simulink model "ENV_hardcoded"  (R2024b)
settings: Solver=FixedStepDiscrete  StartTime=0.0  StopTime=10.0  FixedStep=0.001  RelTol=1e-3
libraries: stm32blockslib x54, canmsglib x29, simulink x7, stm32f4xxblockslib x1
(part 2 of 5)

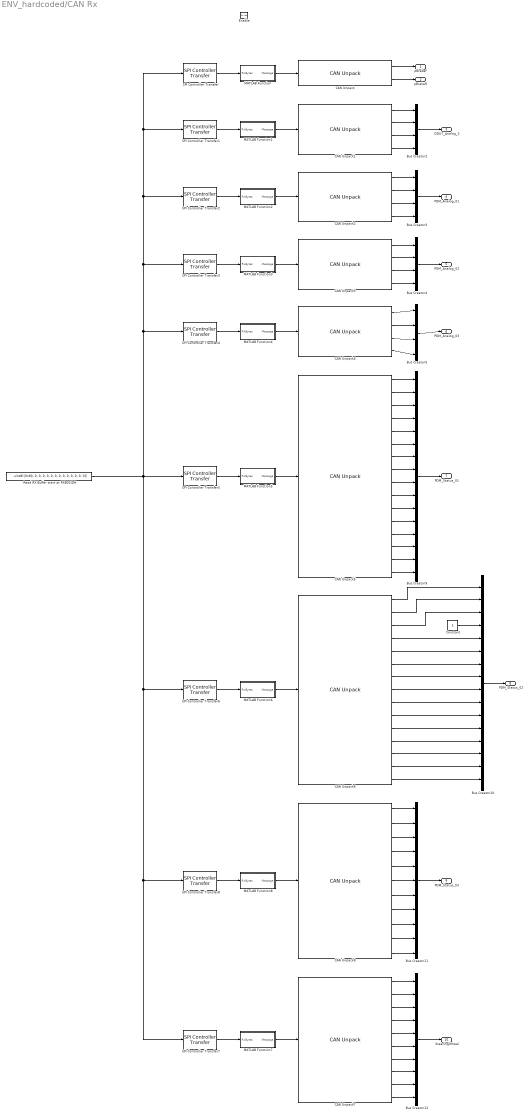
== system ENV_hardcoded/CAN Rx ==
  Enable : EnablePort
  Bus Creator10 : BusCreator  Inputs=16  OutDataTypeStr=Bus: PDM_Status_2
  Bus Creator11 : BusCreator  Inputs=11  OutDataTypeStr=Bus: PDM_Status_3
  Bus Creator12 : BusCreator  Inputs=10  OutDataTypeStr=Bus: SteeringWheelBus
  Bus Creator2 : BusCreator  Inputs=4  OutDataTypeStr=Bus: DDU7_Analoge_2
  Bus Creator3 : BusCreator  Inputs=4  OutDataTypeStr=Bus: PDM_Analoge_1
  Bus Creator4 : BusCreator  Inputs=4  OutDataTypeStr=Bus: PDM_Analoge_2
  Bus Creator5 : BusCreator  Inputs=4  OutDataTypeStr=Bus: PDM_Analoge_3
  Bus Creator9 : BusCreator  Inputs=16  OutDataTypeStr=Bus: PDM_Status_1
  CAN Unpack : canmsglib/CAN Unpack  CANdbFile=C:\Users\William\Downloads\VCUSTM32\BaselineControls\CAN\CAN3_baseline.dbc  MsgList=DDU7_Analoge_1  MsgName=DDU7_Analoge_1  MsgIDType=Standard (11-bit identifier)  MsgIdentifier=2000  MsgLength=8  SignalInfo={'pBrakeF','0','16','LE','signed','Standard','0','0.005','0','-163.84','163.835';'pBrakeR','16','16','LE','signed','Standard','0','0.005','0','-163.84','163.835'}  IDPort=off  TimestampPort=off  ErrorPort=off  RemotePort=off  LengthPort=off  StatusPort=off  ApplyMinMax=off
      settings: LibrarySourceBlock=stmutilitieslib/CAN Unpack  DataFormat=CANdb specified signals
  CAN Unpack1 : canmsglib/CAN Unpack  CANdbFile=C:\Users\William\Downloads\VCUSTM32\BaselineControls\CAN\CAN3_baseline.dbc  MsgList=DDU7_Analoge_2  MsgName=DDU7_Analoge_2  MsgIDType=Standard (11-bit identifier)  MsgIdentifier=2001  MsgLength=8  SignalInfo={'NDisplayNumberDDU7','48','8','LE','unsigned','Standard','0','1','0','0','255';'VSteeringAngle','32','16','LE','unsigned','Standard','0','0.1','0','0','6553.5';'VThrottlePedal1','0','16','LE','unsigned','Standard','0','0.1','0','0','6553.5';'VThrottlePedal2','16','16','LE','unsigned','Standard','0','0.1','0','0','6553.5'}  IDPort=off  TimestampPort=off  ErrorPort=off  RemotePort=off  LengthPort=off  StatusPort=off  ApplyMinMax=off
      settings: LibrarySourceBlock=stmutilitieslib/CAN Unpack  DataFormat=CANdb specified signals
  CAN Unpack2 : canmsglib/CAN Unpack  CANdbFile=C:\Users\William\Downloads\VCUSTM32\BaselineControls\CAN\CAN3_baseline.dbc  MsgList=PDM_Analog_01  MsgName=PDM_Analog_01  MsgIDType=Standard (11-bit identifier)  MsgIdentifier=1540  MsgLength=8  SignalInfo={'C1P14_AnalogInput03','32','10','LE','unsigned','Standard','0','0.005','0','0','5.115';'C1P15_AnalogInput04','48','10','LE','unsigned','Standard','0','0.005','0','0','5.115';'C2P15_AnalogInput01','0','10','LE','unsigned','Standard','0','0.005','0','0','5.115';'C2P16_AnalogInput02','16','10','LE','unsigned','Standard','0','0.005','0','0','5.115'}  IDPort=off  TimestampPort=off  ErrorPort=off  RemotePort=off  LengthPort=off  StatusPort=off  ApplyMinMax=off
      settings: LibrarySourceBlock=stmutilitieslib/CAN Unpack  DataFormat=CANdb specified signals
  CAN Unpack3 : canmsglib/CAN Unpack  CANdbFile=C:\Users\William\Downloads\VCUSTM32\BaselineControls\CAN\CAN3_baseline.dbc  MsgList=PDM_Analog_02  MsgName=PDM_Analog_02  MsgIDType=Standard (11-bit identifier)  MsgIdentifier=1541  MsgLength=8  SignalInfo={'C1P05_AnalogInput07','32','10','LE','unsigned','Standard','0','0.005','0','0','5.115';'C1P06_AnalogInput08','48','10','LE','unsigned','Standard','0','0.005','0','0','5.115';'C1P27_AnalogInput05','0','10','LE','unsigned','Standard','0','0.005','0','0','5.115';'C1P29_AnalogInput06','16','10','LE','unsigned','Standard','0','0.005','0','0','5.115'}  IDPort=off  TimestampPort=off  ErrorPort=off  RemotePort=off  LengthPort=off  StatusPort=off  ApplyMinMax=off
      settings: LibrarySourceBlock=stmutilitieslib/CAN Unpack  DataFormat=CANdb specified signals
  CAN Unpack4 : canmsglib/CAN Unpack  CANdbFile=C:\Users\William\Downloads\VCUSTM32\BaselineControls\CAN\CAN3_baseline.dbc  MsgList=PDM_Analog_03  MsgName=PDM_Analog_03  MsgIDType=Standard (11-bit identifier)  MsgIdentifier=1542  MsgLength=8  SignalInfo={'C1P18_AnalogInput09','0','10','LE','unsigned','Standard','0','0.005','0','-Inf','Inf';'C1P19_AnalogInput10','16','10','LE','unsigned','Standard','0','0.005','0','-Inf','Inf';'C1P32_AnalogInput11','32','10','LE','unsigned','Standard','0','0.005','0','0','5.115';'C1P35_AnalogInput12','48','10','LE','unsigned','Standard','0','0.005','0','0','5.115'}  IDPort=off  TimestampPort=off  ErrorPort=off  RemotePort=off  LengthPort=off  StatusPort=off  ApplyMinMax=off
      settings: LibrarySourceBlock=stmutilitieslib/CAN Unpack  DataFormat=CANdb specified signals
  CAN Unpack5 : canmsglib/CAN Unpack  CANdbFile=C:\Users\William\Downloads\VCUSTM32\BaselineControls\CAN\CAN3_baseline.dbc  MsgList=PDM_Status_01  MsgName=PDM_Status_01  MsgIDType=Standard (11-bit identifier)  MsgIdentifier=1537  MsgLength=8  SignalInfo={'C1P01_Status','0','3','LE','signed','Standard','0','1','0','-4','3';'C1P02_Status','3','3','LE','signed','Standard','0','1','0','-4','3';'C1P03_Status','8','3','LE','signed','Standard','0','1','0','-Inf','Inf';'C1P04_Status','11','3','LE','signed','Standard','0','1','0','-Inf','Inf';'C1P07_Status','16','3','LE','signed','Standard','0','1','0','-4','3';'C1P11_Status','19','3','LE','signed','Standard','0','1','0','-Inf','Inf';'C1P12_Status','24','3','LE','signed','Standard','0','1','0','-Inf','Inf';'C1P13_Status','27','3','LE','signed','Standard','0','1','0','-Inf','Inf';'C1P25_Status','32','3','LE','signed','Standard','0','1','0','-Inf','Inf';'C1P26_Status','35','3','LE','signed','Standard','0','1','0','-Inf','Inf';'C1P28_Status','40','3','LE','signed','Standard','0','1','0','-Inf','Inf';'C1P30_Status','43','3','LE','signed','Standard','0','1','0','-Inf','Inf';'C1P31_Status','48','3','LE','signed','Standard','0','1','0','-Inf','Inf';'C1P33_Status','51','3','LE','signed','Standard','0','1','0','-Inf','Inf';'C1P34_Status','56','3','LE','signed','Standard','0','1','0','-Inf','Inf';'C1P36_Status','59','3','LE','signed','Standard','0','1','0','-Inf','Inf'}  IDPort=off  TimestampPort=off  ErrorPort=off  RemotePort=off  LengthPort=off  StatusPort=off  ApplyMinMax=off
      settings: LibrarySourceBlock=stmutilitieslib/CAN Unpack  DataFormat=CANdb specified signals
  CAN Unpack6 : canmsglib/CAN Unpack  CANdbFile=C:\Users\William\Downloads\VCUSTM32\BaselineControls\CAN\CAN3_baseline.dbc  MsgList=PDM_Status_02  MsgName=PDM_Status_02  MsgIDType=Standard (11-bit identifier)  MsgIdentifier=1538  MsgLength=8  SignalInfo={'C1P37_Status','0','3','LE','signed','Standard','0','1','0','-Inf','Inf';'C1P38_Status','3','3','LE','signed','Standard','0','1','0','-Inf','Inf';'C2P01_Status','8','3','LE','signed','Standard','0','1','0','-Inf','Inf';'C2P03_Status','11','3','LE','signed','Standard','0','1','0','-Inf','Inf';'C2P04_Status','19','3','LE','signed','Standard','0','1','0','-Inf','Inf';'C2P05_Status','24','3','LE','signed','Standard','0','1','0','-Inf','Inf';'C2P13_Status','27','3','LE','signed','Standard','0','1','0','-Inf','Inf';'C2P25_Status','32','3','LE','signed','Standard','0','1','0','-Inf','Inf';'C2P26_Status','35','3','LE','signed','Standard','0','1','0','-Inf','Inf';'C2P27_Status','40','3','LE','signed','Standard','0','1','0','-Inf','Inf';'C2P28_Status','43','3','LE','signed','Standard','0','1','0','-Inf','Inf';'C2P29_Status','48','3','LE','signed','Standard','0','1','0','-Inf','Inf';'C2P30_Status','51','3','LE','signed','Standard','0','1','0','-Inf','Inf';'C2P31_Status','56','3','LE','signed','Standard','0','1','0','-Inf','Inf';'C2P33_Status','59','3','LE','signed','Standard','0','1','0','-Inf','Inf'}  IDPort=off  TimestampPort=off  ErrorPort=off  RemotePort=off  LengthPort=off  StatusPort=off  ApplyMinMax=off
      settings: LibrarySourceBlock=stmutilitieslib/CAN Unpack  DataFormat=CANdb specified signals
  CAN Unpack7 : canmsglib/CAN Unpack  CANdbFile=C:\Users\William\Downloads\VCUSTM32\BaselineControls\CAN\CAN3_baseline.dbc  MsgList=SteeringWheel  MsgName=SteeringWheel  MsgIDType=Standard (11-bit identifier)  MsgIdentifier=801  MsgLength=6  SignalInfo={'BSteeringWheelButton1','0','1','LE','unsigned','Standard','0','1','0','0','1';'BSteeringWheelButton2','1','1','LE','unsigned','Standard','0','1','0','0','1';'BSteeringWheelButton3','2','1','LE','unsigned','Standard','0','1','0','0','1';'BSteeringWheelButton4','3','1','LE','unsigned','Standard','0','1','0','0','1';'BSteeringWheelButton5','4','1','LE','unsigned','Standard','0','1','0','0','1';'BSteeringWheelButton6','5','1','LE','unsigned','Standard','0','1','0','0','1';'BSteeringWheelButton7','6','1','LE','unsigned','Standard','0','1','0','0','1';'BSteeringWheelButton8','7','1','LE','unsigned','Standard','0','1','0','0','1';'VRegenPaddle1','16','16','LE','unsigned','Standard','0','0.001','0','0','65.535';'VRegenPaddle2','32','16','LE','unsigned','Standard','0','0.001','0','0','65.535'}  IDPort=off  TimestampPort=off  ErrorPort=off  RemotePort=off  LengthPort=off  StatusPort=off  ApplyMinMax=off
      settings: LibrarySourceBlock=stmutilitieslib/CAN Unpack  DataFormat=CANdb specified signals
  CAN Unpack8 : canmsglib/CAN Unpack  CANdbFile=C:\Users\William\Downloads\VCUSTM32\BaselineControls\CAN\CAN3_baseline.dbc  MsgList=PDM_Status_03  MsgName=PDM_Status_03  MsgIDType=Standard (11-bit identifier)  MsgIdentifier=1539  MsgLength=8  SignalInfo={'C1P16_Digital','46','3','LE','signed','Standard','0','1','0','-Inf','Inf';'C1P17_Digital','49','3','LE','signed','Standard','0','1','0','-4','3';'C2P17_Digital','40','3','LE','signed','Standard','0','1','0','-Inf','Inf';'C2P18_Digital','43','3','LE','signed','Standard','0','1','0','-Inf','Inf';'C2P35_Status','0','3','LE','signed','Standard','0','1','0','-Inf','Inf';'C2P36_Status','3','3','LE','signed','Standard','0','1','0','-Inf','Inf';'C2P37_Status','8','3','LE','signed','Standard','0','1','0','-Inf','Inf';'C2P38_Status','11','3','LE','signed','Standard','0','1','0','-Inf','Inf';'ILVSystem','16','8','LE','unsigned','Standard','0','1','0','0','255';'TLVSystem','24','8','LE','unsigned','Standard','0','1','0','0','255';'VLVSystem','32','8','LE','unsigned','Standard','0','0.1','0','0','25.5'}  IDPort=off  TimestampPort=off  ErrorPort=off  RemotePort=off  LengthPort=off  StatusPort=off  ApplyMinMax=off
      settings: LibrarySourceBlock=stmutilitieslib/CAN Unpack  DataFormat=CANdb specified signals
  Constant : Constant
  MATLAB Function : MATLAB Function  TreatAsAtomicUnit=on
  MATLAB Function1 : MATLAB Function  TreatAsAtomicUnit=on
  MATLAB Function2 : MATLAB Function  TreatAsAtomicUnit=on
  MATLAB Function3 : MATLAB Function  TreatAsAtomicUnit=on
  MATLAB Function4 : MATLAB Function  TreatAsAtomicUnit=on
  MATLAB Function5 : MATLAB Function  TreatAsAtomicUnit=on
  MATLAB Function6 : MATLAB Function  TreatAsAtomicUnit=on
  MATLAB Function7 : MATLAB Function  TreatAsAtomicUnit=on
  MATLAB Function8 : MATLAB Function  TreatAsAtomicUnit=on
  Read RX Buffer start at RXB0SIDH : Constant  Value=uint8([0x90, 0, 0, 0, 0, 0, 0, 0, 0, 0, 0, 0, 0, 0])
  SPI Controller Transfer : stm32blockslib/SPI Controller Transfer  Priority=1  SPIModuleSelect=SPI1  ClockPolarity=Low  ClockPhase=1 Edge  SPIModule=uint32(0)  Mode=Master  BusSpeed=uint32(1000000)  FirstBitToTransfer=Most significant bit (MSB)  ClockMode=0  BlockFunction=Transfer  EnableRegisterAddress=off  RegisterAddress=0  OutputDataType=uint8  OutputDataLength=1  OutputStatus=off  BlockingMode=off  Timeout=0.01  DataBits=8  UseCustomSSPin=Explicit GPIO calls  ActiveLowSSPin=Active low  Port_Select=GPIOA  Pin=4
      settings: LibrarySourceBlock=stm32h7xxblockslib/SPI Controller Transfer
  SPI Controller Transfer1 : stm32blockslib/SPI Controller Transfer  Priority=2  SPIModuleSelect=SPI1  ClockPolarity=Low  ClockPhase=1 Edge  SPIModule=uint32(0)  Mode=Master  BusSpeed=uint32(1000000)  FirstBitToTransfer=Most significant bit (MSB)  ClockMode=0  BlockFunction=Transfer  EnableRegisterAddress=off  RegisterAddress=0  OutputDataType=uint8  OutputDataLength=1  OutputStatus=off  BlockingMode=off  Timeout=0.01  DataBits=8  UseCustomSSPin=Explicit GPIO calls  ActiveLowSSPin=Active low  Port_Select=GPIOA  Pin=4
      settings: LibrarySourceBlock=stm32h7xxblockslib/SPI Controller Transfer
  SPI Controller Transfer2 : stm32blockslib/SPI Controller Transfer  Priority=3  SPIModuleSelect=SPI1  ClockPolarity=Low  ClockPhase=1 Edge  SPIModule=uint32(0)  Mode=Master  BusSpeed=uint32(1000000)  FirstBitToTransfer=Most significant bit (MSB)  ClockMode=0  BlockFunction=Transfer  EnableRegisterAddress=off  RegisterAddress=0  OutputDataType=uint8  OutputDataLength=1  OutputStatus=off  BlockingMode=off  Timeout=0.01  DataBits=8  UseCustomSSPin=Explicit GPIO calls  ActiveLowSSPin=Active low  Port_Select=GPIOA  Pin=4
      settings: LibrarySourceBlock=stm32h7xxblockslib/SPI Controller Transfer
  SPI Controller Transfer3 : stm32blockslib/SPI Controller Transfer  Priority=4  SPIModuleSelect=SPI1  ClockPolarity=Low  ClockPhase=1 Edge  SPIModule=uint32(0)  Mode=Master  BusSpeed=uint32(1000000)  FirstBitToTransfer=Most significant bit (MSB)  ClockMode=0  BlockFunction=Transfer  EnableRegisterAddress=off  RegisterAddress=0  OutputDataType=uint8  OutputDataLength=1  OutputStatus=off  BlockingMode=off  Timeout=0.01  DataBits=8  UseCustomSSPin=Explicit GPIO calls  ActiveLowSSPin=Active low  Port_Select=GPIOA  Pin=4
      settings: LibrarySourceBlock=stm32h7xxblockslib/SPI Controller Transfer
  SPI Controller Transfer4 : stm32blockslib/SPI Controller Transfer  Priority=5  SPIModuleSelect=SPI1  ClockPolarity=Low  ClockPhase=1 Edge  SPIModule=uint32(0)  Mode=Master  BusSpeed=uint32(1000000)  FirstBitToTransfer=Most significant bit (MSB)  ClockMode=0  BlockFunction=Transfer  EnableRegisterAddress=off  RegisterAddress=0  OutputDataType=uint8  OutputDataLength=1  OutputStatus=off  BlockingMode=off  Timeout=0.01  DataBits=8  UseCustomSSPin=Explicit GPIO calls  ActiveLowSSPin=Active low  Port_Select=GPIOA  Pin=4
      settings: LibrarySourceBlock=stm32h7xxblockslib/SPI Controller Transfer
  SPI Controller Transfer5 : stm32blockslib/SPI Controller Transfer  Priority=6  SPIModuleSelect=SPI1  ClockPolarity=Low  ClockPhase=1 Edge  SPIModule=uint32(0)  Mode=Master  BusSpeed=uint32(1000000)  FirstBitToTransfer=Most significant bit (MSB)  ClockMode=0  BlockFunction=Transfer  EnableRegisterAddress=off  RegisterAddress=0  OutputDataType=uint8  OutputDataLength=1  OutputStatus=off  BlockingMode=off  Timeout=0.01  DataBits=8  UseCustomSSPin=Explicit GPIO calls  ActiveLowSSPin=Active low  Port_Select=GPIOA  Pin=4
      settings: LibrarySourceBlock=stm32h7xxblockslib/SPI Controller Transfer
  SPI Controller Transfer6 : stm32blockslib/SPI Controller Transfer  Priority=7  SPIModuleSelect=SPI1  ClockPolarity=Low  ClockPhase=1 Edge  SPIModule=uint32(0)  Mode=Master  BusSpeed=uint32(1000000)  FirstBitToTransfer=Most significant bit (MSB)  ClockMode=0  BlockFunction=Transfer  EnableRegisterAddress=off  RegisterAddress=0  OutputDataType=uint8  OutputDataLength=1  OutputStatus=off  BlockingMode=off  Timeout=0.01  DataBits=8  UseCustomSSPin=Explicit GPIO calls  ActiveLowSSPin=Active low  Port_Select=GPIOA  Pin=4
      settings: LibrarySourceBlock=stm32h7xxblockslib/SPI Controller Transfer
  SPI Controller Transfer7 : stm32blockslib/SPI Controller Transfer  Priority=8  SPIModuleSelect=SPI1  ClockPolarity=Low  ClockPhase=1 Edge  SPIModule=uint32(0)  Mode=Master  BusSpeed=uint32(1000000)  FirstBitToTransfer=Most significant bit (MSB)  ClockMode=0  BlockFunction=Transfer  EnableRegisterAddress=off  RegisterAddress=0  OutputDataType=uint8  OutputDataLength=1  OutputStatus=off  BlockingMode=off  Timeout=0.01  DataBits=8  UseCustomSSPin=Explicit GPIO calls  ActiveLowSSPin=Active low  Port_Select=GPIOA  Pin=4
      settings: LibrarySourceBlock=stm32h7xxblockslib/SPI Controller Transfer
  SPI Controller Transfer8 : stm32blockslib/SPI Controller Transfer  Priority=6  SPIModuleSelect=SPI1  ClockPolarity=Low  ClockPhase=1 Edge  SPIModule=uint32(0)  Mode=Master  BusSpeed=uint32(1000000)  FirstBitToTransfer=Most significant bit (MSB)  ClockMode=0  BlockFunction=Transfer  EnableRegisterAddress=off  RegisterAddress=0  OutputDataType=uint8  OutputDataLength=1  OutputStatus=off  BlockingMode=off  Timeout=0.01  DataBits=8  UseCustomSSPin=Explicit GPIO calls  ActiveLowSSPin=Active low  Port_Select=GPIOA  Pin=4
      settings: LibrarySourceBlock=stm32h7xxblockslib/SPI Controller Transfer
  pBrakeF : Outport  OutDataTypeStr=double
  pBrakeR : Outport  Port=2  OutDataTypeStr=double
  DDU7_Analog_2 : Outport  Port=3
  PDM_Analog_01 : Outport  Port=4
  PDM_Analog_02 : Outport  Port=5
  PDM_Analog_03 : Outport  Port=6
  PDM_Status_01 : Outport  Port=7
  PDM_Status_02 : Outport  Port=8
  PDM_Status_03 : Outport  Port=9
  SteeringWheel : Outport  Port=10
  wires:
  SPI Controller Transfer/1 -> MATLAB Function/1(RxBytes)
  MATLAB Function/1(Message) -> CAN Unpack/1
  SPI Controller Transfer1/1 -> MATLAB Function1/1(RxBytes)
  MATLAB Function1/1(Message) -> CAN Unpack1/1
  Read RX Buffer start at RXB0SIDH/1 -> SPI Controller Transfer/1, SPI Controller Transfer1/1, SPI Controller Transfer2/1, SPI Controller Transfer3/1, SPI Controller Transfer4/1, SPI Controller Transfer8/1, SPI Controller Transfer7/1, SPI Controller Transfer6/1, SPI Controller Transfer5/1
  CAN Unpack/1 -> pBrakeF/1
  CAN Unpack/2 -> pBrakeR/1
  CAN Unpack1/2 -> Bus Creator2/2
  CAN Unpack1/1 -> Bus Creator2/1
  CAN Unpack1/3 -> Bus Creator2/3
  CAN Unpack1/4 -> Bus Creator2/4
  CAN Unpack2/2 -> Bus Creator3/2
  SPI Controller Transfer2/1 -> MATLAB Function2/1(RxBytes)
  CAN Unpack2/3 -> Bus Creator3/3
  CAN Unpack2/4 -> Bus Creator3/4
  MATLAB Function2/1(Message) -> CAN Unpack2/1
  CAN Unpack2/1 -> Bus Creator3/1
  CAN Unpack3/3 -> Bus Creator4/3
  MATLAB Function3/1(Message) -> CAN Unpack3/1
  CAN Unpack3/1 -> Bus Creator4/1
  CAN Unpack3/4 -> Bus Creator4/4
  SPI Controller Transfer3/1 -> MATLAB Function3/1(RxBytes)
  CAN Unpack3/2 -> Bus Creator4/2
  CAN Unpack4/1 -> Bus Creator5/1
  MATLAB Function4/1(Message) -> CAN Unpack4/1
  SPI Controller Transfer4/1 -> MATLAB Function4/1(RxBytes)
  CAN Unpack4/4 -> Bus Creator5/4
  CAN Unpack4/3 -> Bus Creator5/3
  CAN Unpack4/2 -> Bus Creator5/2
  CAN Unpack5/2 -> Bus Creator9/2
  MATLAB Function5/1(Message) -> CAN Unpack5/1
  CAN Unpack5/1 -> Bus Creator9/1
  SPI Controller Transfer5/1 -> MATLAB Function5/1(RxBytes)
  CAN Unpack5/3 -> Bus Creator9/3
  CAN Unpack5/4 -> Bus Creator9/4
  CAN Unpack5/8 -> Bus Creator9/8
  CAN Unpack5/6 -> Bus Creator9/6
  CAN Unpack5/7 -> Bus Creator9/7
  CAN Unpack5/5 -> Bus Creator9/5
  CAN Unpack5/12 -> Bus Creator9/12
  CAN Unpack5/10 -> Bus Creator9/10
  CAN Unpack5/11 -> Bus Creator9/11
  CAN Unpack5/9 -> Bus Creator9/9
  CAN Unpack5/16 -> Bus Creator9/16
  CAN Unpack5/14 -> Bus Creator9/14
  CAN Unpack5/15 -> Bus Creator9/15
  CAN Unpack5/13 -> Bus Creator9/13
  CAN Unpack6/12 -> Bus Creator10/13
  CAN Unpack6/10 -> Bus Creator10/11
  CAN Unpack6/9 -> Bus Creator10/10
  CAN Unpack6/11 -> Bus Creator10/12
  CAN Unpack6/5 -> Bus Creator10/6
  CAN Unpack6/6 -> Bus Creator10/7
  CAN Unpack6/7 -> Bus Creator10/8
  CAN Unpack6/8 -> Bus Creator10/9
  SPI Controller Transfer6/1 -> MATLAB Function6/1(RxBytes)
  CAN Unpack6/2 -> Bus Creator10/2
  MATLAB Function6/1(Message) -> CAN Unpack6/1
  CAN Unpack6/13 -> Bus Creator10/14
  CAN Unpack6/3 -> Bus Creator10/3
  CAN Unpack6/1 -> Bus Creator10/1
  CAN Unpack6/14 -> Bus Creator10/15
  CAN Unpack6/4 -> Bus Creator10/5
  CAN Unpack6/15 -> Bus Creator10/16
  CAN Unpack7/1 -> Bus Creator12/1
  CAN Unpack7/3 -> Bus Creator12/3
  CAN Unpack7/4 -> Bus Creator12/4
  SPI Controller Transfer7/1 -> MATLAB Function7/1(RxBytes)
  CAN Unpack7/8 -> Bus Creator12/8
  CAN Unpack7/10 -> Bus Creator12/10
  CAN Unpack7/9 -> Bus Creator12/9
  CAN Unpack7/5 -> Bus Creator12/5
  CAN Unpack7/7 -> Bus Creator12/7
  MATLAB Function7/1(Message) -> CAN Unpack7/1
  CAN Unpack7/2 -> Bus Creator12/2
  CAN Unpack7/6 -> Bus Creator12/6
  Bus Creator10/1 -> PDM_Status_02/1
  Constant/1 -> Bus Creator10/4
  Bus Creator2/1 -> DDU7_Analog_2/1
  Bus Creator3/1 -> PDM_Analog_01/1
  Bus Creator4/1 -> PDM_Analog_02/1
  Bus Creator5/1 -> PDM_Analog_03/1
  Bus Creator9/1 -> PDM_Status_01/1
  Bus Creator12/1 -> SteeringWheel/1
  SPI Controller Transfer8/1 -> MATLAB Function8/1(RxBytes)
  MATLAB Function8/1(Message) -> CAN Unpack8/1
  CAN Unpack8/1 -> Bus Creator11/1
  CAN Unpack8/2 -> Bus Creator11/2
  CAN Unpack8/3 -> Bus Creator11/3
  CAN Unpack8/4 -> Bus Creator11/4
  CAN Unpack8/5 -> Bus Creator11/5
  CAN Unpack8/6 -> Bus Creator11/6
  CAN Unpack8/7 -> Bus Creator11/7
  CAN Unpack8/8 -> Bus Creator11/8
  CAN Unpack8/9 -> Bus Creator11/9
  CAN Unpack8/10 -> Bus Creator11/10
  CAN Unpack8/11 -> Bus Creator11/11
  Bus Creator11/1 -> PDM_Status_03/1

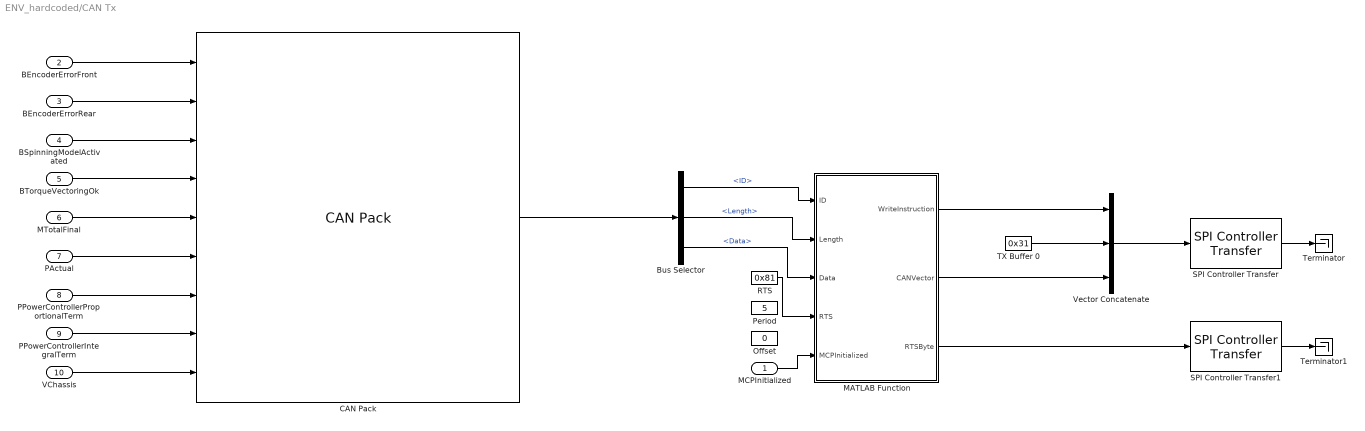
== system ENV_hardcoded/CAN Tx ==
  MCPInitialized : Inport  SampleTime=.001
  BEncoderErrorFront : Inport  Port=2  SampleTime=.001
  BEncoderErrorRear : Inport  Port=3  SampleTime=.001
  BSpinningModelActivated : Inport  Port=4  SampleTime=.001
  BTorqueVectoringOk : Inport  Port=5  SampleTime=.001
  MTotalFinal : Inport  Port=6  SampleTime=.001
  PActual : Inport  Port=7  SampleTime=.001
  PPowerControllerProportionalTerm : Inport  Port=8  SampleTime=.001
  PPowerControllerIntegralTerm : Inport  Port=9  SampleTime=.001
  VChassis : Inport  Port=10  SampleTime=.001
  Bus Selector : BusSelector  OutputSignals=ID,Length,Data
  CAN Pack : canmsglib/CAN Pack  CANdbFile=C:\Users\William\Downloads\VCUSTM32\BaselineControls\CAN\CAN3_baseline.dbc  MsgList=Etas_Signals_01  MsgName=Etas_Signals_01  MsgIDType=Standard (11-bit identifier)  MsgIdentifier=2022  CANIDInput=off  MsgLength=8  Remote=off  ApplyMinMax=off  BusOutput=on  SignalInfo={'BEncoderErrorFront','62','1','LE','unsigned','Standard','0','1','0','0','1';'BEncoderErrorRear','63','1','LE','unsigned','Standard','0','1','0','0','1';'BSpinningModelActivated','60','1','LE','unsigned','Standard','0','1','0','0','1';'BTorqueVectoringOk','61','1','LE','unsigned','Standard','0','1','0','0','1';'MTotalFinal','11','14','LE','signed','Standard','0','0.1','300','-Inf','Inf';'PActual','25','14','LE','signed','Standard','0','0.01','30','-51.92','111.91';'PPowerControlerProportionalTerm','0','11','LE','signed','Standard','0','0.01','0','-10.24','10.23';'PPowerControllerIntergralTerm','49','11','LE','signed','Standard','0','0.01','0','-10.24','10.23';'vChassis','39','10','LE','signed','Standard','0','0.1','0','-51.2','51.1'}
      settings: LibrarySourceBlock=stmutilitieslib/CAN Pack  DataFormat=CANdb specified signals
  MATLAB Function : MATLAB Function  TreatAsAtomicUnit=on
  Offset : Constant  Value=0  OutDataTypeStr=uint16  SampleTime=.001
  Period : Constant  Value=5  OutDataTypeStr=uint16  SampleTime=.001
  RTS : Constant  Value=0x81  OutDataTypeStr=uint8  SampleTime=.001
  SPI Controller Transfer : stm32blockslib/SPI Controller Transfer  Priority=1  SPIModuleSelect=SPI1  ClockPolarity=Low  ClockPhase=1 Edge  SPIModule=uint32(0)  Mode=Master  BusSpeed=uint32(1000000)  FirstBitToTransfer=Most significant bit (MSB)  ClockMode=0  BlockFunction=Transfer  EnableRegisterAddress=off  RegisterAddress=0  OutputDataType=uint8  OutputDataLength=1  OutputStatus=off  BlockingMode=off  Timeout=0.01  DataBits=8  UseCustomSSPin=Explicit GPIO calls  ActiveLowSSPin=Active low  Port_Select=GPIOA  Pin=4
      settings: LibrarySourceBlock=stm32h7xxblockslib/SPI Controller Transfer
  SPI Controller Transfer1 : stm32blockslib/SPI Controller Transfer  Priority=2  SPIModuleSelect=SPI1  ClockPolarity=Low  ClockPhase=1 Edge  SPIModule=uint32(0)  Mode=Master  BusSpeed=uint32(1000000)  FirstBitToTransfer=Most significant bit (MSB)  ClockMode=0  BlockFunction=Transfer  EnableRegisterAddress=off  RegisterAddress=0  OutputDataType=uint8  OutputDataLength=1  OutputStatus=off  BlockingMode=off  Timeout=0.01  DataBits=8  UseCustomSSPin=Explicit GPIO calls  ActiveLowSSPin=Active low  Port_Select=GPIOA  Pin=4
      settings: LibrarySourceBlock=stm32h7xxblockslib/SPI Controller Transfer
  TX Buffer 0 : Constant  Value=0x31  OutDataTypeStr=uint8  SampleTime=.001
  Terminator : Terminator
  Terminator1 : Terminator
  Vector Concatenate : Concatenate  NumInputs=3
  wires:
  CAN Pack/1 -> Bus Selector/1
  BEncoderErrorFront/1 -> CAN Pack/1
  BTorqueVectoringOk/1 -> CAN Pack/4
  BSpinningModelActivated/1 -> CAN Pack/3
  BEncoderErrorRear/1 -> CAN Pack/2
  MTotalFinal/1 -> CAN Pack/5
  PActual/1 -> CAN Pack/6
  PPowerControllerProportionalTerm/1 -> CAN Pack/7
  PPowerControllerIntegralTerm/1 -> CAN Pack/8
  VChassis/1 -> CAN Pack/9
  RTS/1 -> MATLAB Function/4(RTS)
  Bus Selector/1 -> MATLAB Function/1(ID)  "<ID>"
  Bus Selector/2 -> MATLAB Function/2(Length)  "<Length>"
  Bus Selector/3 -> MATLAB Function/3(Data)  "<Data>"
  MCPInitialized/1 -> MATLAB Function/5(MCPInitialized)
  Vector Concatenate/1 -> SPI Controller Transfer/1
  MATLAB Function/1(WriteInstruction) -> Vector Concatenate/1
  SPI Controller Transfer1/1 -> Terminator1/1
  TX Buffer 0/1 -> Vector Concatenate/2
  SPI Controller Transfer/1 -> Terminator/1
  MATLAB Function/3(RTSByte) -> SPI Controller Transfer1/1
  MATLAB Function/2(CANVector) -> Vector Concatenate/3

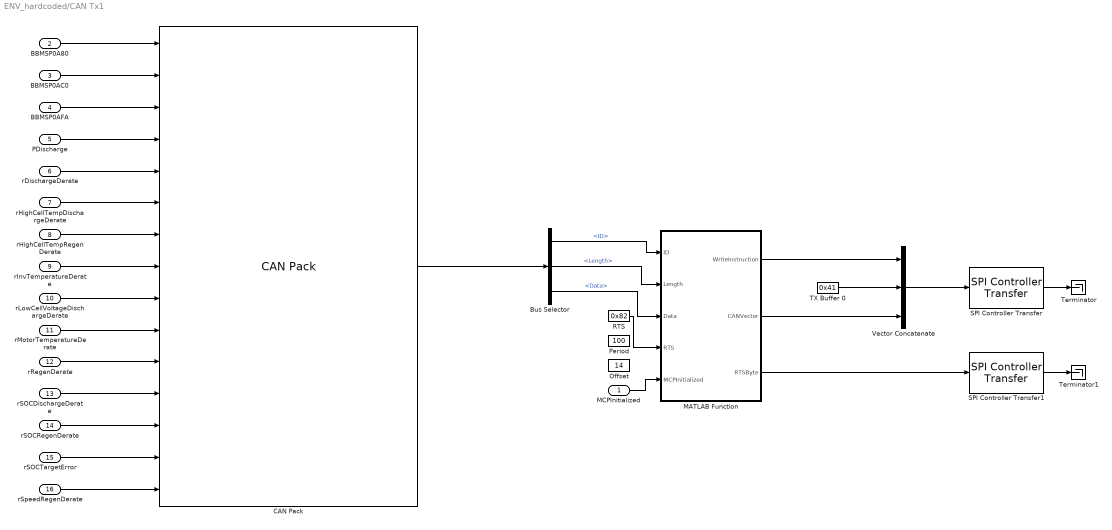
== system ENV_hardcoded/CAN Tx1 ==
  MCPInitialized : Inport  SampleTime=.001
  BBMSP0A80 : Inport  Port=2  SampleTime=.001
  BBMSP0AC0 : Inport  Port=3  SampleTime=.001
  BBMSP0AFA : Inport  Port=4  SampleTime=.001
  PDischarge : Inport  Port=5  SampleTime=.001
  rDischargeDerate : Inport  Port=6  SampleTime=.001
  rHighCellTempDischargeDerate : Inport  Port=7  SampleTime=.001
  rHighCellTempRegenDerate : Inport  Port=8  SampleTime=.001
  rInvTemperatureDerate : Inport  Port=9  SampleTime=.001
  rLowCellVoltageDischargeDerate : Inport  Port=10  SampleTime=.001
  rMotorTemperatureDerate : Inport  Port=11  SampleTime=.001
  rRegenDerate : Inport  Port=12  SampleTime=.001
  rSOCDischargeDerate : Inport  Port=13  SampleTime=.001
  rSOCRegenDerate : Inport  Port=14  SampleTime=.001
  rSOCTargetError : Inport  Port=15  SampleTime=.001
  rSpeedRegenDerate : Inport  Port=16  SampleTime=.001
  Bus Selector : BusSelector  OutputSignals=ID,Length,Data
  CAN Pack : canmsglib/CAN Pack  CANdbFile=C:\Users\William\Downloads\VCUSTM32\BaselineControls\CAN\CAN3_baseline.dbc  MsgList=Etas_Signals_02  MsgName=Etas_Signals_02  MsgIDType=Standard (11-bit identifier)  MsgIdentifier=2023  CANIDInput=off  MsgLength=8  Remote=off  ApplyMinMax=off  BusOutput=on  SignalInfo={'BBMSP0A80','0','1','LE','unsigned','Standard','0','1','0','0','1';'BBMSP0AC0','1','1','LE','unsigned','Standard','0','1','0','0','1';'BBMSP0AFA','2','1','LE','unsigned','Standard','0','1','0','0','1';'PDischarge','43','8','LE','unsigned','Standard','0','1','0','0','255';'rDischargeDerate','35','4','LE','unsigned','Standard','0','0.1','0','0','1.5';'rHighCellTempDischargeDerate','3','4','LE','unsigned','Standard','0','0.1','0','0','1.5';'rHighCellTempRegenDerate','7','4','LE','unsigned','Standard','0','0.1','0','0','1.5';'rInvTemperatureDerate','11','4','LE','unsigned','Standard','0','0.1','0','0','1.5';'rLowCellVoltageDischargeDerate','19','4','LE','unsigned','Standard','0','0.1','0','0','1.5';'rMotorTemperatureDerate','15','4','LE','unsigned','Standard','0','0.1','0','0','1.5';'rRegenDerate','39','4','LE','unsigned','Standard','0','0.1','0','0','1.5';'rSOCDischargeDerate','23','4','LE','unsigned','Standard','0','0.1','0','0','1.5';'rSOCRegenDerate','27','4','LE','unsigned','Standard','0','0.1','0','0','1.5';'rSOCTargetError','51','13','LE','signed','Standard','0','0.001','0','-4.096','4.095';'rSpeedRegenDerate','31','4','LE','unsigned','Standard','0','0.1','0','0','1.5'}
      settings: LibrarySourceBlock=stmutilitieslib/CAN Pack  DataFormat=CANdb specified signals
  MATLAB Function : MATLAB Function  TreatAsAtomicUnit=on
  Offset : Constant  Value=14  OutDataTypeStr=uint16  SampleTime=.001
  Period : Constant  Value=100  OutDataTypeStr=uint16  SampleTime=.001
  RTS : Constant  Value=0x82  OutDataTypeStr=uint8  SampleTime=.001
  SPI Controller Transfer : stm32blockslib/SPI Controller Transfer  Priority=1  SPIModuleSelect=SPI1  ClockPolarity=Low  ClockPhase=1 Edge  SPIModule=uint32(0)  Mode=Master  BusSpeed=uint32(1000000)  FirstBitToTransfer=Most significant bit (MSB)  ClockMode=0  BlockFunction=Transfer  EnableRegisterAddress=off  RegisterAddress=0  OutputDataType=uint8  OutputDataLength=1  OutputStatus=off  BlockingMode=off  Timeout=0.01  DataBits=8  UseCustomSSPin=Explicit GPIO calls  ActiveLowSSPin=Active low  Port_Select=GPIOA  Pin=4
      settings: LibrarySourceBlock=stm32h7xxblockslib/SPI Controller Transfer
  SPI Controller Transfer1 : stm32blockslib/SPI Controller Transfer  Priority=2  SPIModuleSelect=SPI1  ClockPolarity=Low  ClockPhase=1 Edge  SPIModule=uint32(0)  Mode=Master  BusSpeed=uint32(1000000)  FirstBitToTransfer=Most significant bit (MSB)  ClockMode=0  BlockFunction=Transfer  EnableRegisterAddress=off  RegisterAddress=0  OutputDataType=uint8  OutputDataLength=1  OutputStatus=off  BlockingMode=off  Timeout=0.01  DataBits=8  UseCustomSSPin=Explicit GPIO calls  ActiveLowSSPin=Active low  Port_Select=GPIOA  Pin=4
      settings: LibrarySourceBlock=stm32h7xxblockslib/SPI Controller Transfer
  TX Buffer 0 : Constant  Value=0x41  OutDataTypeStr=uint8  SampleTime=.001
  Terminator : Terminator
  Terminator1 : Terminator
  Vector Concatenate : Concatenate  NumInputs=3
  wires:
  BBMSP0AC0/1 -> CAN Pack/2
  BBMSP0A80/1 -> CAN Pack/1
  BBMSP0AFA/1 -> CAN Pack/3
  PDischarge/1 -> CAN Pack/4
  rDischargeDerate/1 -> CAN Pack/5
  rHighCellTempDischargeDerate/1 -> CAN Pack/6
  rHighCellTempRegenDerate/1 -> CAN Pack/7
  rInvTemperatureDerate/1 -> CAN Pack/8
  rLowCellVoltageDischargeDerate/1 -> CAN Pack/9
  rSOCDischargeDerate/1 -> CAN Pack/12
  rSOCRegenDerate/1 -> CAN Pack/13
  rRegenDerate/1 -> CAN Pack/11
  rSOCTargetError/1 -> CAN Pack/14
  rSpeedRegenDerate/1 -> CAN Pack/15
  rMotorTemperatureDerate/1 -> CAN Pack/10
  MATLAB Function/3(RTSByte) -> SPI Controller Transfer1/1
  Bus Selector/3 -> MATLAB Function/3(Data)  "<Data>"
  RTS/1 -> MATLAB Function/4(RTS)
  MATLAB Function/1(WriteInstruction) -> Vector Concatenate/1
  Vector Concatenate/1 -> SPI Controller Transfer/1
  Bus Selector/2 -> MATLAB Function/2(Length)  "<Length>"
  SPI Controller Transfer1/1 -> Terminator1/1
  SPI Controller Transfer/1 -> Terminator/1
  TX Buffer 0/1 -> Vector Concatenate/2
  CAN Pack/1 -> Bus Selector/1
  Bus Selector/1 -> MATLAB Function/1(ID)  "<ID>"
  MCPInitialized/1 -> MATLAB Function/5(MCPInitialized)
  MATLAB Function/2(CANVector) -> Vector Concatenate/3

== system ENV_hardcoded/CAN Tx10 ==
  MCPInitialized : Inport  SampleTime=.001
  VDamperPotentiometerRL : Inport  Port=2
  VDamperPotentiometerRR : Inport  Port=3
  Bus Selector : BusSelector  OutputSignals=ID,Length,Data
  CAN Pack : canmsglib/CAN Pack  CANdbFile=C:\Users\William\Downloads\VCUSTM32\BaselineControls\CAN\CAN3_baseline.dbc  MsgList=Etas_Signals_11  MsgName=Etas_Signals_11  MsgIDType=Standard (11-bit identifier)  MsgIdentifier=1796  CANIDInput=off  MsgLength=8  Remote=off  ApplyMinMax=off  BusOutput=on  SignalInfo={'VDamperPotentiometerRL','0','10','LE','unsigned','Standard','0','0.005','0','0','5.115';'VDamperPotentiometerRR','16','10','LE','unsigned','Standard','0','0.005','0','0','5.115'}
      settings: LibrarySourceBlock=stmutilitieslib/CAN Pack  DataFormat=CANdb specified signals
  MATLAB Function : MATLAB Function  TreatAsAtomicUnit=on
  Offset : Constant  Value=8  OutDataTypeStr=uint16  SampleTime=.001
  Period : Constant  Value=100  OutDataTypeStr=uint16  SampleTime=.001
  RTS : Constant  Value=0x82  OutDataTypeStr=uint8  SampleTime=.001
  SPI Controller Transfer : stm32blockslib/SPI Controller Transfer  Priority=1  SPIModuleSelect=SPI1  ClockPolarity=Low  ClockPhase=1 Edge  SPIModule=uint32(0)  Mode=Master  BusSpeed=uint32(1000000)  FirstBitToTransfer=Most significant bit (MSB)  ClockMode=0  BlockFunction=Transfer  EnableRegisterAddress=off  RegisterAddress=0  OutputDataType=uint8  OutputDataLength=1  OutputStatus=off  BlockingMode=off  Timeout=0.01  DataBits=8  UseCustomSSPin=Explicit GPIO calls  ActiveLowSSPin=Active low  Port_Select=GPIOA  Pin=4
      settings: LibrarySourceBlock=stm32h7xxblockslib/SPI Controller Transfer
  SPI Controller Transfer1 : stm32blockslib/SPI Controller Transfer  Priority=2  SPIModuleSelect=SPI1  ClockPolarity=Low  ClockPhase=1 Edge  SPIModule=uint32(0)  Mode=Master  BusSpeed=uint32(1000000)  FirstBitToTransfer=Most significant bit (MSB)  ClockMode=0  BlockFunction=Transfer  EnableRegisterAddress=off  RegisterAddress=0  OutputDataType=uint8  OutputDataLength=1  OutputStatus=off  BlockingMode=off  Timeout=0.01  DataBits=8  UseCustomSSPin=Explicit GPIO calls  ActiveLowSSPin=Active low  Port_Select=GPIOA  Pin=4
      settings: LibrarySourceBlock=stm32h7xxblockslib/SPI Controller Transfer
  TX Buffer 0 : Constant  Value=0x41  OutDataTypeStr=uint8  SampleTime=.001
  Terminator : Terminator
  Terminator1 : Terminator
  Vector Concatenate : Concatenate  NumInputs=3
  wires:
  VDamperPotentiometerRR/1 -> CAN Pack/2
  VDamperPotentiometerRL/1 -> CAN Pack/1
  RTS/1 -> MATLAB Function/4(RTS)
  MATLAB Function/1(WriteInstruction) -> Vector Concatenate/1
  TX Buffer 0/1 -> Vector Concatenate/2
  SPI Controller Transfer1/1 -> Terminator1/1
  MATLAB Function/2(CANVector) -> Vector Concatenate/3
  Bus Selector/2 -> MATLAB Function/2(Length)  "<Length>"
  Bus Selector/3 -> MATLAB Function/3(Data)  "<Data>"
  Vector Concatenate/1 -> SPI Controller Transfer/1
  MCPInitialized/1 -> MATLAB Function/5(MCPInitialized)
  Bus Selector/1 -> MATLAB Function/1(ID)  "<ID>"
  CAN Pack/1 -> Bus Selector/1
  SPI Controller Transfer/1 -> Terminator/1
  MATLAB Function/3(RTSByte) -> SPI Controller Transfer1/1

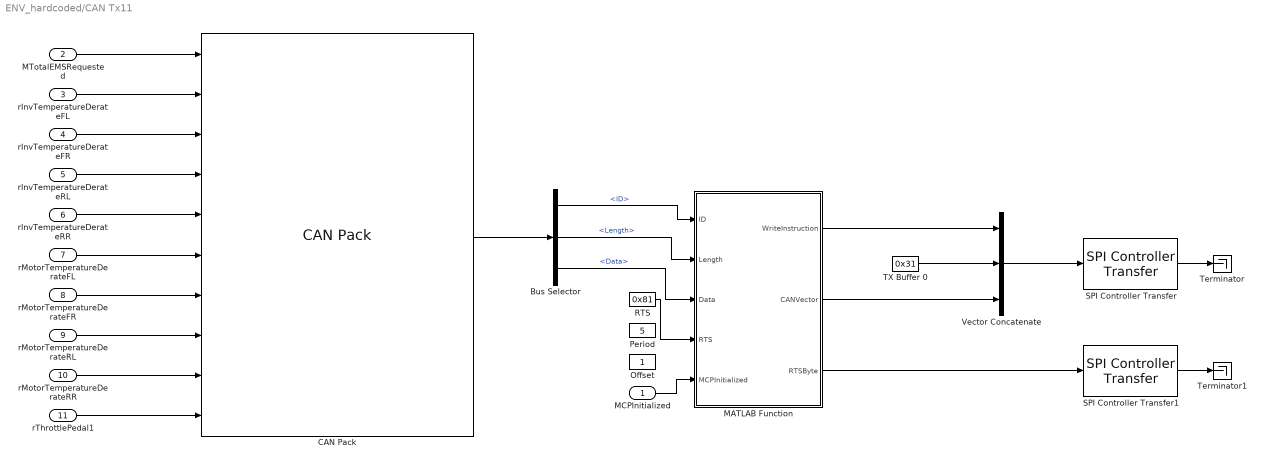
== system ENV_hardcoded/CAN Tx11 ==
  MCPInitialized : Inport  SampleTime=.001
  MTotalEMSRequested : Inport  Port=2
  rInvTemperatureDerateFL : Inport  Port=3
  rInvTemperatureDerateFR : Inport  Port=4
  rInvTemperatureDerateRL : Inport  Port=5
  rInvTemperatureDerateRR : Inport  Port=6
  rMotorTemperatureDerateFL : Inport  Port=7
  rMotorTemperatureDerateFR : Inport  Port=8
  rMotorTemperatureDerateRL : Inport  Port=9
  rMotorTemperatureDerateRR : Inport  Port=10
  rThrottlePedal1 : Inport  Port=11
  Bus Selector : BusSelector  OutputSignals=ID,Length,Data
  CAN Pack : canmsglib/CAN Pack  CANdbFile=C:\Users\William\Downloads\VCUSTM32\BaselineControls\CAN\CAN3_baseline.dbc  MsgList=Etas_Signals_12  MsgName=Etas_Signals_12  MsgIDType=Standard (11-bit identifier)  MsgIdentifier=2039  CANIDInput=off  MsgLength=8  Remote=off  ApplyMinMax=off  BusOutput=on  SignalInfo={'MTotalEMSRequested','32','14','LE','signed','Standard','0','0.1','300','-519.2','1119.1';'rInvTemperatureDerateFL','4','4','LE','unsigned','Standard','0','0.1','0','0','1.5';'rInvTemperatureDerateFR','8','4','LE','unsigned','Standard','0','0.1','0','0','1.5';'rInvTemperatureDerateRL','12','4','LE','unsigned','Standard','0','0.1','0','0','1.5';'rInvTemperatureDerateRR','16','4','LE','unsigned','Standard','0','0.1','0','0','1.5';'rMotorTemperatureDerateFL','20','4','LE','unsigned','Standard','0','0.1','0','0','1.5';'rMotorTemperatureDerateFR','24','4','LE','unsigned','Standard','0','0.1','0','0','1.5';'rMotorTemperatureDerateRL','28','4','LE','unsigned','Standard','0','0.1','0','-Inf','Inf';'rMotorTemperatureDerateRR','0','4','LE','unsigned','Standard','0','0.1','0','0','1.5';'rThrottlePedal1','46','10','LE','unsigned','Standard','0','0.1','0','0','102.3'}
      settings: LibrarySourceBlock=stmutilitieslib/CAN Pack  DataFormat=CANdb specified signals
  MATLAB Function : MATLAB Function  TreatAsAtomicUnit=on
  Offset : Constant  OutDataTypeStr=uint16  SampleTime=.001
  Period : Constant  Value=5  OutDataTypeStr=uint16  SampleTime=.001
  RTS : Constant  Value=0x81  OutDataTypeStr=uint8  SampleTime=.001
  SPI Controller Transfer : stm32blockslib/SPI Controller Transfer  Priority=1  SPIModuleSelect=SPI1  ClockPolarity=Low  ClockPhase=1 Edge  SPIModule=uint32(0)  Mode=Master  BusSpeed=uint32(1000000)  FirstBitToTransfer=Most significant bit (MSB)  ClockMode=0  BlockFunction=Transfer  EnableRegisterAddress=off  RegisterAddress=0  OutputDataType=uint8  OutputDataLength=1  OutputStatus=off  BlockingMode=off  Timeout=0.01  DataBits=8  UseCustomSSPin=Explicit GPIO calls  ActiveLowSSPin=Active low  Port_Select=GPIOA  Pin=4
      settings: LibrarySourceBlock=stm32h7xxblockslib/SPI Controller Transfer
  SPI Controller Transfer1 : stm32blockslib/SPI Controller Transfer  Priority=2  SPIModuleSelect=SPI1  ClockPolarity=Low  ClockPhase=1 Edge  SPIModule=uint32(0)  Mode=Master  BusSpeed=uint32(1000000)  FirstBitToTransfer=Most significant bit (MSB)  ClockMode=0  BlockFunction=Transfer  EnableRegisterAddress=off  RegisterAddress=0  OutputDataType=uint8  OutputDataLength=1  OutputStatus=off  BlockingMode=off  Timeout=0.01  DataBits=8  UseCustomSSPin=Explicit GPIO calls  ActiveLowSSPin=Active low  Port_Select=GPIOA  Pin=4
      settings: LibrarySourceBlock=stm32h7xxblockslib/SPI Controller Transfer
  TX Buffer 0 : Constant  Value=0x31  OutDataTypeStr=uint8  SampleTime=.001
  Terminator : Terminator
  Terminator1 : Terminator
  Vector Concatenate : Concatenate  NumInputs=3
  wires:
  rInvTemperatureDerateFL/1 -> CAN Pack/2
  MTotalEMSRequested/1 -> CAN Pack/1
  rInvTemperatureDerateFR/1 -> CAN Pack/3
  rInvTemperatureDerateRL/1 -> CAN Pack/4
  rInvTemperatureDerateRR/1 -> CAN Pack/5
  rMotorTemperatureDerateFL/1 -> CAN Pack/6
  rMotorTemperatureDerateFR/1 -> CAN Pack/7
  rMotorTemperatureDerateRL/1 -> CAN Pack/8
  rMotorTemperatureDerateRR/1 -> CAN Pack/9
  rThrottlePedal1/1 -> CAN Pack/10
  RTS/1 -> MATLAB Function/4(RTS)
  MATLAB Function/1(WriteInstruction) -> Vector Concatenate/1
  TX Buffer 0/1 -> Vector Concatenate/2
  SPI Controller Transfer1/1 -> Terminator1/1
  MATLAB Function/2(CANVector) -> Vector Concatenate/3
  Bus Selector/2 -> MATLAB Function/2(Length)  "<Length>"
  Bus Selector/3 -> MATLAB Function/3(Data)  "<Data>"
  Vector Concatenate/1 -> SPI Controller Transfer/1
  MCPInitialized/1 -> MATLAB Function/5(MCPInitialized)
  Bus Selector/1 -> MATLAB Function/1(ID)  "<ID>"
  CAN Pack/1 -> Bus Selector/1
  SPI Controller Transfer/1 -> Terminator/1
  MATLAB Function/3(RTSByte) -> SPI Controller Transfer1/1

== system ENV_hardcoded/CAN Tx12 ==
  MCPInitialized : Inport  SampleTime=.001
  nMotorFL : Inport  Port=2
  nMotorFR : Inport  Port=3
  nMotorRL : Inport  Port=4
  nMotorRR : Inport  Port=5
  Bus Selector : BusSelector  OutputSignals=ID,Length,Data
  CAN Pack : canmsglib/CAN Pack  CANdbFile=C:\Users\William\Downloads\VCUSTM32\BaselineControls\CAN\CAN3_baseline.dbc  MsgList=Etas_Signals_13  MsgName=Etas_Signals_13  MsgIDType=Standard (11-bit identifier)  MsgIdentifier=2008  CANIDInput=off  MsgLength=8  Remote=off  ApplyMinMax=off  BusOutput=on  SignalInfo={'nMotorFL','0','16','LE','signed','Standard','0','1','0','-32768','32767';'nMotorFR','16','16','LE','signed','Standard','0','1','0','-32768','32767';'nMotorRL','32','16','LE','signed','Standard','0','1','0','-32768','32767';'nMotorRR','48','16','LE','signed','Standard','0','1','0','-32768','32767'}
      settings: LibrarySourceBlock=stmutilitieslib/CAN Pack  DataFormat=CANdb specified signals
  MATLAB Function : MATLAB Function  TreatAsAtomicUnit=on
  Offset : Constant  OutDataTypeStr=uint16  SampleTime=.001
  Period : Constant  Value=10  OutDataTypeStr=uint16  SampleTime=.001
  RTS : Constant  Value=0x82  OutDataTypeStr=uint8  SampleTime=.001
  SPI Controller Transfer : stm32blockslib/SPI Controller Transfer  Priority=1  SPIModuleSelect=SPI1  ClockPolarity=Low  ClockPhase=1 Edge  SPIModule=uint32(0)  Mode=Master  BusSpeed=uint32(1000000)  FirstBitToTransfer=Most significant bit (MSB)  ClockMode=0  BlockFunction=Transfer  EnableRegisterAddress=off  RegisterAddress=0  OutputDataType=uint8  OutputDataLength=1  OutputStatus=off  BlockingMode=off  Timeout=0.01  DataBits=8  UseCustomSSPin=Explicit GPIO calls  ActiveLowSSPin=Active low  Port_Select=GPIOA  Pin=4
      settings: LibrarySourceBlock=stm32h7xxblockslib/SPI Controller Transfer
  SPI Controller Transfer1 : stm32blockslib/SPI Controller Transfer  Priority=2  SPIModuleSelect=SPI1  ClockPolarity=Low  ClockPhase=1 Edge  SPIModule=uint32(0)  Mode=Master  BusSpeed=uint32(1000000)  FirstBitToTransfer=Most significant bit (MSB)  ClockMode=0  BlockFunction=Transfer  EnableRegisterAddress=off  RegisterAddress=0  OutputDataType=uint8  OutputDataLength=1  OutputStatus=off  BlockingMode=off  Timeout=0.01  DataBits=8  UseCustomSSPin=Explicit GPIO calls  ActiveLowSSPin=Active low  Port_Select=GPIOA  Pin=4
      settings: LibrarySourceBlock=stm32h7xxblockslib/SPI Controller Transfer
  TX Buffer 0 : Constant  Value=0x41  OutDataTypeStr=uint8  SampleTime=.001
  Terminator : Terminator
  Terminator1 : Terminator
  Vector Concatenate : Concatenate  NumInputs=3
  wires:
  nMotorFR/1 -> CAN Pack/2
  nMotorFL/1 -> CAN Pack/1
  nMotorRL/1 -> CAN Pack/3
  nMotorRR/1 -> CAN Pack/4
  Bus Selector/2 -> MATLAB Function/2(Length)  "<Length>"
  Vector Concatenate/1 -> SPI Controller Transfer/1
  Bus Selector/1 -> MATLAB Function/1(ID)  "<ID>"
  SPI Controller Transfer/1 -> Terminator/1
  MATLAB Function/1(WriteInstruction) -> Vector Concatenate/1
  MATLAB Function/3(RTSByte) -> SPI Controller Transfer1/1
  RTS/1 -> MATLAB Function/4(RTS)
  SPI Controller Transfer1/1 -> Terminator1/1
  Bus Selector/3 -> MATLAB Function/3(Data)  "<Data>"
  MATLAB Function/2(CANVector) -> Vector Concatenate/3
  CAN Pack/1 -> Bus Selector/1
  TX Buffer 0/1 -> Vector Concatenate/2
  MCPInitialized/1 -> MATLAB Function/5(MCPInitialized)

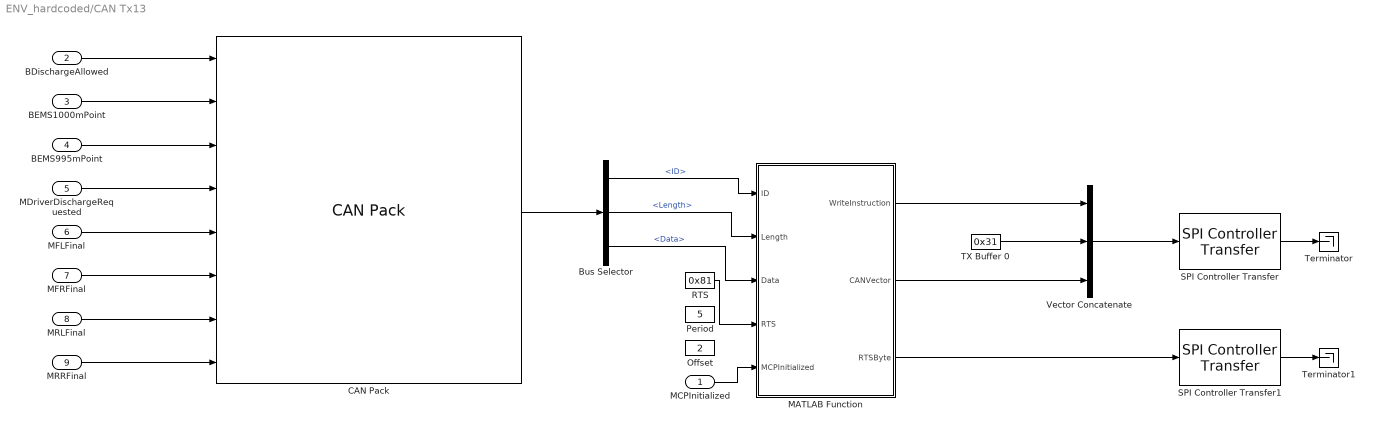
== system ENV_hardcoded/CAN Tx13 ==
  MCPInitialized : Inport  SampleTime=.001
  BDischargeAllowed : Inport  Port=2
  BEMS1000mPoint : Inport  Port=3
  BEMS995mPoint : Inport  Port=4
  MDriverDischargeRequested : Inport  Port=5
  MFLFinal : Inport  Port=6
  MFRFinal : Inport  Port=7
  MRLFinal : Inport  Port=8
  MRRFinal : Inport  Port=9
  Bus Selector : BusSelector  OutputSignals=ID,Length,Data
  CAN Pack : canmsglib/CAN Pack  CANdbFile=C:\Users\William\Downloads\VCUSTM32\BaselineControls\CAN\CAN3_baseline.dbc  MsgList=Etas_Signals_14  MsgName=Etas_Signals_14  MsgIDType=Standard (11-bit identifier)  MsgIdentifier=2009  CANIDInput=off  MsgLength=8  Remote=off  ApplyMinMax=off  BusOutput=on  SignalInfo={'BDischargeAllowed','63','1','LE','unsigned','Standard','0','1','0','0','1';'BEMS1000mPoint','61','1','LE','unsigned','Standard','0','1','0','0','1';'BEMS995mPoint','62','1','LE','unsigned','Standard','0','1','0','0','1';'MDriverDischargeRequested','48','13','LE','unsigned','Standard','0','0.1','0','0','819.1';'MFLFinal','12','12','LE','signed','Standard','0','0.1','50','-154.8','254.7';'MFRFinal','0','12','LE','signed','Standard','0','0.1','50','-154.8','254.7';'MRLFinal','24','12','LE','signed','Standard','0','0.1','50','-154.8','254.7';'MRRFinal','36','12','LE','signed','Standard','0','0.1','50','-154.8','254.7'}
      settings: LibrarySourceBlock=stmutilitieslib/CAN Pack  DataFormat=CANdb specified signals
  MATLAB Function : MATLAB Function  TreatAsAtomicUnit=on
  Offset : Constant  Value=2  OutDataTypeStr=uint16  SampleTime=.001
  Period : Constant  Value=5  OutDataTypeStr=uint16  SampleTime=.001
  RTS : Constant  Value=0x81  OutDataTypeStr=uint8  SampleTime=.001
  SPI Controller Transfer : stm32blockslib/SPI Controller Transfer  Priority=1  SPIModuleSelect=SPI1  ClockPolarity=Low  ClockPhase=1 Edge  SPIModule=uint32(0)  Mode=Master  BusSpeed=uint32(1000000)  FirstBitToTransfer=Most significant bit (MSB)  ClockMode=0  BlockFunction=Transfer  EnableRegisterAddress=off  RegisterAddress=0  OutputDataType=uint8  OutputDataLength=1  OutputStatus=off  BlockingMode=off  Timeout=0.01  DataBits=8  UseCustomSSPin=Explicit GPIO calls  ActiveLowSSPin=Active low  Port_Select=GPIOA  Pin=4
      settings: LibrarySourceBlock=stm32h7xxblockslib/SPI Controller Transfer
  SPI Controller Transfer1 : stm32blockslib/SPI Controller Transfer  Priority=2  SPIModuleSelect=SPI1  ClockPolarity=Low  ClockPhase=1 Edge  SPIModule=uint32(0)  Mode=Master  BusSpeed=uint32(1000000)  FirstBitToTransfer=Most significant bit (MSB)  ClockMode=0  BlockFunction=Transfer  EnableRegisterAddress=off  RegisterAddress=0  OutputDataType=uint8  OutputDataLength=1  OutputStatus=off  BlockingMode=off  Timeout=0.01  DataBits=8  UseCustomSSPin=Explicit GPIO calls  ActiveLowSSPin=Active low  Port_Select=GPIOA  Pin=4
      settings: LibrarySourceBlock=stm32h7xxblockslib/SPI Controller Transfer
  TX Buffer 0 : Constant  Value=0x31  OutDataTypeStr=uint8  SampleTime=.001
  Terminator : Terminator
  Terminator1 : Terminator
  Vector Concatenate : Concatenate  NumInputs=3
  wires:
  BEMS1000mPoint/1 -> CAN Pack/2
  BDischargeAllowed/1 -> CAN Pack/1
  BEMS995mPoint/1 -> CAN Pack/3
  MDriverDischargeRequested/1 -> CAN Pack/4
  MFLFinal/1 -> CAN Pack/5
  MFRFinal/1 -> CAN Pack/6
  MRLFinal/1 -> CAN Pack/7
  MRRFinal/1 -> CAN Pack/8
  CAN Pack/1 -> Bus Selector/1
  SPI Controller Transfer/1 -> Terminator/1
  Bus Selector/1 -> MATLAB Function/1(ID)  "<ID>"
  Bus Selector/3 -> MATLAB Function/3(Data)  "<Data>"
  Vector Concatenate/1 -> SPI Controller Transfer/1
  Bus Selector/2 -> MATLAB Function/2(Length)  "<Length>"
  SPI Controller Transfer1/1 -> Terminator1/1
  MATLAB Function/2(CANVector) -> Vector Concatenate/3
  TX Buffer 0/1 -> Vector Concatenate/2
  MATLAB Function/3(RTSByte) -> SPI Controller Transfer1/1
  RTS/1 -> MATLAB Function/4(RTS)
  MCPInitialized/1 -> MATLAB Function/5(MCPInitialized)
  MATLAB Function/1(WriteInstruction) -> Vector Concatenate/1
